simulink subsystem "rss_MosOpnCirFaltDia"  (R2023a)
settings: Solver=VariableStepAuto  StartTime=0.0  StopTime=10.0  RelTol=1e-3
undefined symbols (not defined in the file): ENM_TYPE_FALT, Gu16_ctMosOpnCirFaltConfCnt_C, Gu16_ctMosOpnCirFaltRcvyCnt_C
libraries: lib_debounce x1, lib_fault_definiteness x1
settings Model: Creator=xiaoqiang.yuan  LastModifiedBy=xiaoqiang.yuan

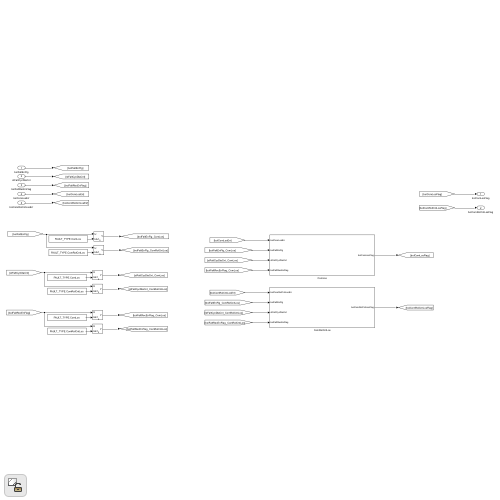
[thumbnail: Simulink's stored preview of the top-level diagram]
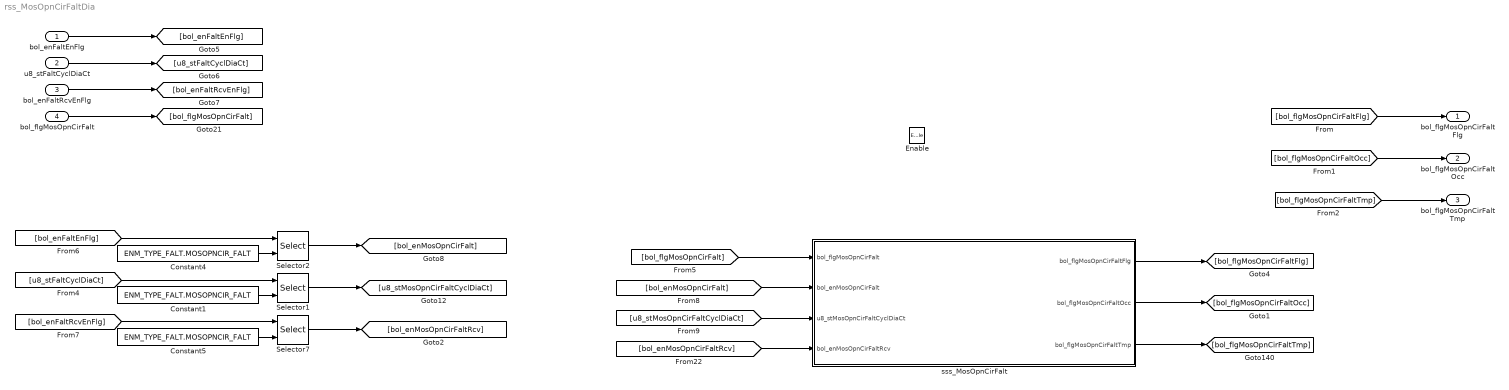
== system rss_MosOpnCirFaltDia ==
  bol_enFaltEnFlg : Inport  OutDataTypeStr=boolean
  u8_stFaltCyclDiaCt : Inport  Port=2  OutDataTypeStr=uint8
  bol_enFaltRcvEnFlg : Inport  Port=3  OutDataTypeStr=boolean
  bol_flgMosOpnCirFalt : Inport  Port=4  OutDataTypeStr=boolean
  Enable : EnablePort
  Constant1 : Constant  Value=ENM_TYPE_FALT.MOSOPNCIR_FALT
  Constant4 : Constant  Value=ENM_TYPE_FALT.MOSOPNCIR_FALT
  Constant5 : Constant  Value=ENM_TYPE_FALT.MOSOPNCIR_FALT
  Selector1 : Selector  IndexMode=Zero-based  InputPortWidth=Cdbl_numFaltDiaNum  IndexOptions=Index vector (port)  Indices=[1 3]  OutputSizes=1
  Selector2 : Selector  IndexMode=Zero-based  InputPortWidth=Cdbl_numFaltDiaNum  IndexOptions=Index vector (port)  Indices=[1 3]  OutputSizes=1
  Selector7 : Selector  IndexMode=Zero-based  InputPortWidth=Cdbl_numFaltDiaNum  IndexOptions=Index vector (port)  Indices=[1 3]  OutputSizes=1
  sss_MosOpnCirFalt : Subsystem
  bol_flgMosOpnCirFaltFlg : Outport  OutDataTypeStr=boolean
  bol_flgMosOpnCirFaltOcc : Outport  Port=2  OutDataTypeStr=boolean
  bol_flgMosOpnCirFaltTmp : Outport  Port=3  OutDataTypeStr=boolean
  wires:
  [bol_flgMosOpnCirFaltFlg] -> bol_flgMosOpnCirFaltFlg/1
  [u8_stFaltCyclDiaCt] -> Selector1/1
  [bol_enFaltEnFlg] -> Selector2/1
  bol_enFaltEnFlg/1 -> [bol_enFaltEnFlg]
  bol_enFaltRcvEnFlg/1 -> [bol_enFaltRcvEnFlg]
  [bol_flgMosOpnCirFalt] -> sss_MosOpnCirFalt/1(bol_flgMosOpnCirFalt)
  Constant1/1 -> Selector1/2
  [u8_stMosOpnCirFaltCyclDiaCt] -> sss_MosOpnCirFalt/3(u8_stMosOpnCirFaltCyclDiaCt)
  [bol_enMosOpnCirFalt] -> sss_MosOpnCirFalt/2(bol_enMosOpnCirFalt)
  Constant4/1 -> Selector2/2
  Constant5/1 -> Selector7/2
  Selector1/1 -> [u8_stMosOpnCirFaltCyclDiaCt]
  bol_flgMosOpnCirFalt/1 -> [bol_flgMosOpnCirFalt]
  Selector7/1 -> [bol_enMosOpnCirFaltRcv]
  [bol_enFaltRcvEnFlg] -> Selector7/1
  Selector2/1 -> [bol_enMosOpnCirFalt]
  [bol_enMosOpnCirFaltRcv] -> sss_MosOpnCirFalt/4(bol_enMosOpnCirFaltRcv)
  u8_stFaltCyclDiaCt/1 -> [u8_stFaltCyclDiaCt]
  sss_MosOpnCirFalt/1(bol_flgMosOpnCirFaltFlg) -> [bol_flgMosOpnCirFaltFlg]
  sss_MosOpnCirFalt/2(bol_flgMosOpnCirFaltOcc) -> [bol_flgMosOpnCirFaltOcc]
  [bol_flgMosOpnCirFaltOcc] -> bol_flgMosOpnCirFaltOcc/1
  [bol_flgMosOpnCirFaltTmp] -> bol_flgMosOpnCirFaltTmp/1
  sss_MosOpnCirFalt/3(bol_flgMosOpnCirFaltTmp) -> [bol_flgMosOpnCirFaltTmp]

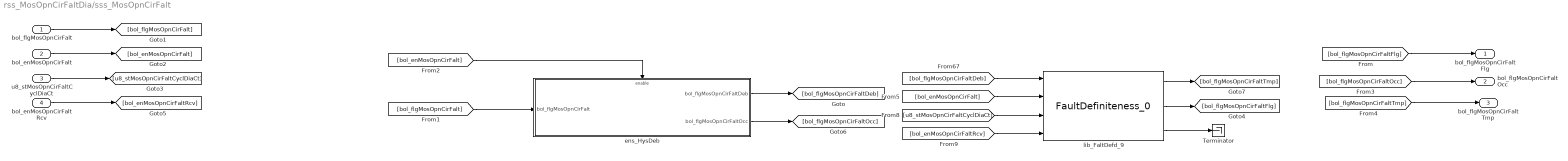
== system rss_MosOpnCirFaltDia/sss_MosOpnCirFalt ==
  bol_flgMosOpnCirFalt : Inport
  bol_enMosOpnCirFalt : Inport  Port=2
  u8_stMosOpnCirFaltCyclDiaCt : Inport  Port=3
  bol_enMosOpnCirFaltRcv : Inport  Port=4
  Terminator : Terminator
  ens_HysDeb : Subsystem
  lib_FaltDefd_9 : lib_fault_definiteness/FaultDefiniteness_0  lb_FaltWaitRecvCnt=Gu16_ctMosOpnCirFaltConfCnt_C
  bol_flgMosOpnCirFaltFlg : Outport
  bol_flgMosOpnCirFaltOcc : Outport  Port=2
  bol_flgMosOpnCirFaltTmp : Outport  Port=3
  wires:
  [bol_flgMosOpnCirFaltTmp] -> bol_flgMosOpnCirFaltTmp/1
  [bol_flgMosOpnCirFaltOcc] -> bol_flgMosOpnCirFaltOcc/1
  ens_HysDeb/2(bol_flgMosOpnCirFaltOcc) -> [bol_flgMosOpnCirFaltOcc]
  lib_FaltDefd_9/1 -> [bol_flgMosOpnCirFaltTmp]
  lib_FaltDefd_9/2 -> [bol_flgMosOpnCirFaltFlg]
  lib_FaltDefd_9/3 -> Terminator/1
  [bol_enMosOpnCirFalt] -> ens_HysDeb/Enable
  [bol_flgMosOpnCirFalt] -> ens_HysDeb/1(bol_flgMosOpnCirFalt)
  ens_HysDeb/1(bol_flgMosOpnCirFaltDeb) -> [bol_flgMosOpnCirFaltDeb]
  bol_enMosOpnCirFaltRcv/1 -> [bol_enMosOpnCirFaltRcv]
  u8_stMosOpnCirFaltCyclDiaCt/1 -> [u8_stMosOpnCirFaltCyclDiaCt]
  bol_enMosOpnCirFalt/1 -> [bol_enMosOpnCirFalt]
  [bol_flgMosOpnCirFaltFlg] -> bol_flgMosOpnCirFaltFlg/1
  bol_flgMosOpnCirFalt/1 -> [bol_flgMosOpnCirFalt]
  [bol_enMosOpnCirFaltRcv] -> lib_FaltDefd_9/4
  [u8_stMosOpnCirFaltCyclDiaCt] -> lib_FaltDefd_9/3
  [bol_enMosOpnCirFalt] -> lib_FaltDefd_9/2
  [bol_flgMosOpnCirFaltDeb] -> lib_FaltDefd_9/1

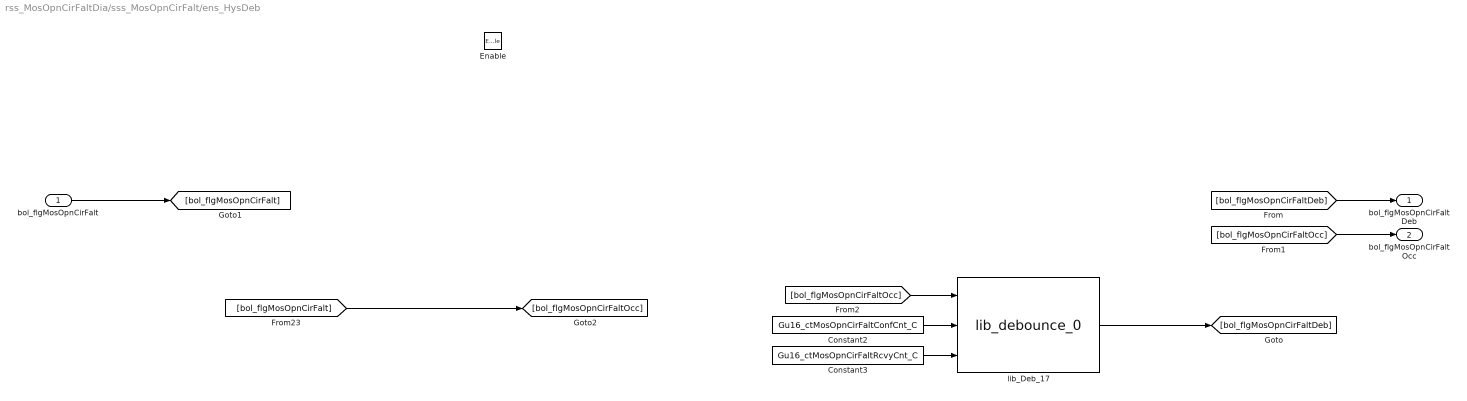
== system rss_MosOpnCirFaltDia/sss_MosOpnCirFalt/ens_HysDeb ==
  bol_flgMosOpnCirFalt : Inport
  Enable : EnablePort
  Constant2 : Constant  Value=Gu16_ctMosOpnCirFaltConfCnt_C
  Constant3 : Constant  Value=Gu16_ctMosOpnCirFaltRcvyCnt_C
  lib_Deb_17 : lib_debounce/lib_debounce_0
  bol_flgMosOpnCirFaltDeb : Outport
  bol_flgMosOpnCirFaltOcc : Outport  Port=2
  wires:
  [bol_flgMosOpnCirFaltOcc] -> lib_Deb_17/1
  [bol_flgMosOpnCirFalt] -> [bol_flgMosOpnCirFaltOcc]
  [bol_flgMosOpnCirFaltOcc] -> bol_flgMosOpnCirFaltOcc/1
  lib_Deb_17/1 -> [bol_flgMosOpnCirFaltDeb]
  bol_flgMosOpnCirFalt/1 -> [bol_flgMosOpnCirFalt]
  [bol_flgMosOpnCirFaltDeb] -> bol_flgMosOpnCirFaltDeb/1
  Constant3/1 -> lib_Deb_17/3
  Constant2/1 -> lib_Deb_17/2
